simulink subsystem "GantryRobotSubsystem"  (R2024a)
settings: Solver=VariableStepAuto  StartTime=0.0  StopTime=10.0  RelTol=1e-3
model mask{DOF=3DOF, configAxis=XYZ, heightColumn=0.4, widthColumn=0.05, positionColumn1=[-0.5,-0.5,0], positionColumn2=[0.5,-0.5,0], positionColumn3=[-0.5,0.5,0], positionColumn4=[0.5,0.5,0], systemGuideX=Rail-block, strokeXMax=1, widthGuideX=0.05, diaScrewX=0.05, widthXMount=0.1, typeInertiaGuideX=Calculate from Geometry, densityGuideX=2700, massGuideX=0.1, COMGuideX=[0 0 0], MOIGuideX=[0.01 0.01 0.01], POIGuideX=[0 0 0], typeInertiaCarriageX=Calculate from Geometry, densityCarriageX=2700, massCarriageX=0.1, COMCarriageX=[0 0 0], MOICarriageX=[0.01 0.01 0.01], POICarriageX=[0 0 0], colorGuideX=[0.7 0.6 0.4], colorCarriageX=[0.5 0.5 0.9], systemGuideY=Rail-block, strokeYMax=1, widthGuideY=0.05, diaScrewY=0.05, widthYMount=0.05, typeInertiaGuideY=Calculate from Geometry, densityGuideY=2700, massGuideY=0.1, COMGuideY=[0 0 0], MOIGuideY=[0.01 0.01 0.01], POIGuideY=[0 0 0], typeInertiaCarriageY=Calculate from Geometry, densityCarriageY=2700, massCarriageY=0.1, COMCarriageY=[0 0 0], MOICarriageY=[0.01 0.01 0.01], POICarriageY=[0 0 0], colorGuideY=[0.7 0.6 0.4], colorCarriageY=[0.5 0.5 0.9], systemGuideZ=Rail-block, strokeZMax=1, widthGuideZ=0.05, diaScrewZ=0.05, shiftZAxisDown=0.02, widthZMount=0.05, typeInertiaGuideZ=Calculate from Geometry, densityGuideZ=2700, massGuideZ=0.1, COMGuideZ=[0 0 0], MOIGuideZ=[0.01 0.01 0.01], POIGuideZ=[0 0 0], typeInertiaCarriageZ=Calculate from Geometry, densityCarriageZ=2700, massCarriageZ=0.1, COMCarriageZ=[0 0 0], MOICarriageZ=[0.01 0.01 0.01], POICarriageZ=[0 0 0], colorGuideZ=[0.7 0.6 0.4], colorCarriageZ=[0.5 0.5 0.9]}
  mask prompts: DOF "Degrees of freedom"; configAxis "Axis configurations"; heightColumn "Column height (m)"; widthColumn "Column width (m)"; positionColumn1 "Column 1 position (m)"; positionColumn2 "Column 2 position (m)"; positionColumn3 "Column 3 position (m)"; positionColumn4 "Column 4 position (m)"; systemGuideX "Guide system"; strokeXMax "Maximum stroke (m)"; widthGuideX "Guide width (m)"; diaScrewX "Screw diameter (m)"; widthXMount "Mount width (m)"; typeInertiaGuideX "Inertia type"; densityGuideX "Density (kg/m^3)"; massGuideX "Mass (kg)"; COMGuideX "Center of mass (m)"; MOIGuideX "Moments of inertia (kg*m^2)"; POIGuideX "Products of inertia (kg*m^2)"; typeInertiaCarriageX "Inertia type"; densityCarriageX "Density (kg/m^3)"; massCarriageX "Mass (kg)"; COMCarriageX "Center of mass (m)"; MOICarriageX "Moments of inertia (kg*m^2)"; POICarriageX "Products of inertia (kg*m^2)"; colorGuideX "Linear guide color"; colorCarriageX "Carriage color"; systemGuideY "Guide system"; strokeYMax "Maximum stroke (m)"; widthGuideY "Guide width (m)"; diaScrewY "Screw diameter (m)"; widthYMount "Mount width (m)"; typeInertiaGuideY "Inertia type"; densityGuideY "Density (kg/m^3)"; massGuideY "Mass (kg)"; COMGuideY "Center of mass (m)"; MOIGuideY "Moments of inertia (kg*m^2)"; POIGuideY "Products of inertia (kg*m^2)"; typeInertiaCarriageY "Inertia type"; densityCarriageY "Density (kg/m^3)"; massCarriageY "Mass (kg)"; COMCarriageY "Center of mass (m)"; MOICarriageY "Moments of inertia (kg*m^2)"; POICarriageY "Products of inertia (kg*m^2)"; colorGuideY "Linear guide color"; colorCarriageY "Carriage color"; systemGuideZ "Guide system"; strokeZMax "Maximum stroke (m)"; widthGuideZ "Guide width (m)"; diaScrewZ "Screw diameter (m)"; shiftZAxisDown "Downward shift of Z-axis (m)"; widthZMount "Mount width (m)"; typeInertiaGuideZ "Inertia type"; densityGuideZ "Density (kg/m^3)"; massGuideZ "Mass (kg)"; COMGuideZ "Center of mass (m)"; MOIGuideZ "Moments of inertia (kg*m^2)"; POIGuideZ "Products of inertia (kg*m^2)"; typeInertiaCarriageZ "Inertia type"; densityCarriageZ "Density (kg/m^3)"; massCarriageZ "Mass (kg)"; COMCarriageZ "Center of mass (m)"; MOICarriageZ "Moments of inertia (kg*m^2)"; POICarriageZ "Products of inertia (kg*m^2)"; colorGuideZ "Linear guide color"; colorCarriageZ "Carriage color"
undefined symbols (not defined in the file): X, Y, Z
libraries: sm_lib x92, CartesianLib x46, nesl_utility x38
(part 1 of 4)
settings Model: Creator=abirdas  LastModifiedBy=abirdas

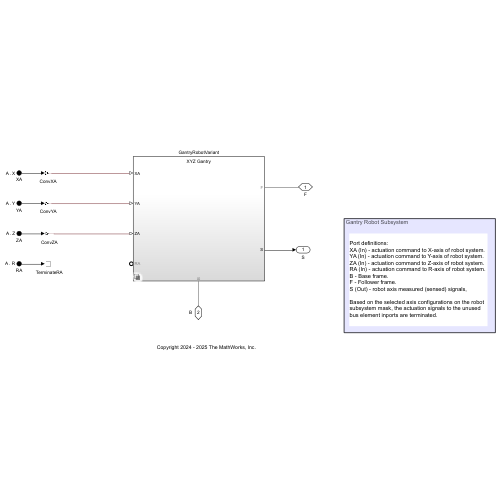
[thumbnail: Simulink's stored preview of the top-level diagram]
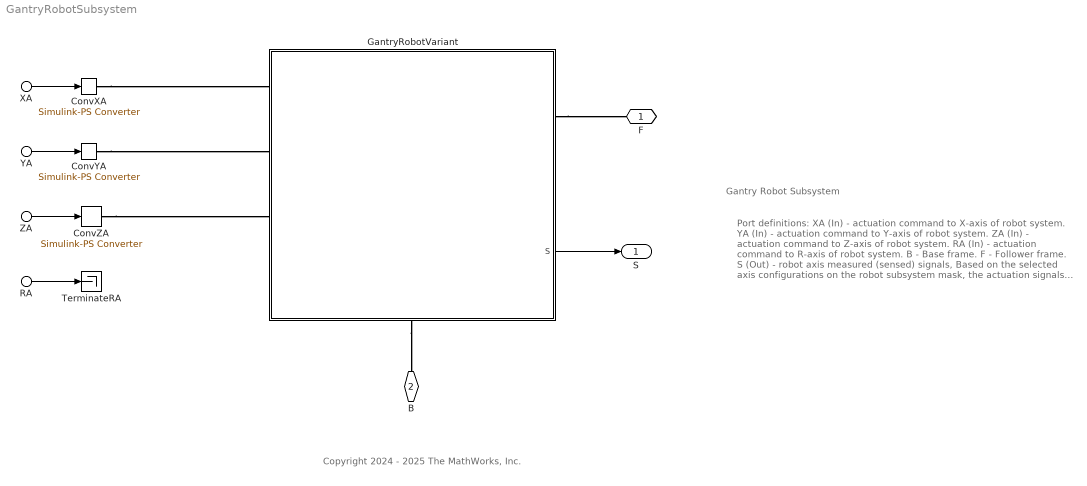
== system GantryRobotSubsystem ==
  note: Port definitions:
      | XA (In) - actuation command to X-axis of robot system.
      | YA (In) - actuation command to Y-axis of robot system.
      | ZA (In) - actuation command to Z-axis of robot system.
      | RA (In) - actuation command to R-axis of robot system.
      | B - Base frame.
      | F - Follower frame.
      | S (Out) - robot axis measured (sensed) signals,
      |
      | Based on the selected axis configurations on the robot subsystem mask, the actuation signals to the unused bus element inports are terminated.
  note: Gantry Robot Subsystem
  note: Copyright 2024 - 2025 The MathWorks, Inc.
  XA : Inport  PortName=A  Element=X
  YA : Inport  PortName=A  Element=Y
  ZA : Inport  PortName=A  Element=Z
  RA : Inport  PortName=A  Element=R
  ConvXA : nesl_utility/Simulink-PS Converter  PhysicalDomain=network_engine_domain  SubClassName=ps_input  LeftPortType=input  RightPortType=output  PseudoPeriodic=off  Frequencies=[]  NoiseDistribution=none  NoiseParameters=[]  Unit=N  AffineConversion=off  FilteringAndDerivatives=provide  SimscapeFilterOrder=1  InputFilterTimeConstant=0.001  UdotUserProvided=0
  ConvYA : nesl_utility/Simulink-PS Converter  PhysicalDomain=network_engine_domain  SubClassName=ps_input  LeftPortType=input  RightPortType=output  PseudoPeriodic=off  Frequencies=[]  NoiseDistribution=none  NoiseParameters=[]  Unit=N  AffineConversion=off  FilteringAndDerivatives=provide  SimscapeFilterOrder=1  InputFilterTimeConstant=0.001  UdotUserProvided=0
  ConvZA : nesl_utility/Simulink-PS Converter  PhysicalDomain=network_engine_domain  SubClassName=ps_input  LeftPortType=input  RightPortType=output  PseudoPeriodic=off  Frequencies=[]  NoiseDistribution=none  NoiseParameters=[]  Unit=N  AffineConversion=off  FilteringAndDerivatives=provide  SimscapeFilterOrder=1  InputFilterTimeConstant=0.001  UdotUserProvided=0
  GantryRobotVariant : Subsystem  Variant=on  VariantControlMode=label  VariantControl=Cartesian Robot  LabelModeActiveChoice=XYZG
      settings: PortSchema="{\"entries\":[{\"content\":{\"sides\":[{\"content\":{\"connectorIds\":[\"LConn1\",\"LConn2\",\"LConn3\",\"LConn4\"]},\"type\":\"ConnectorPlacement.EquallySpacedRectSide\",\"uuid\":\"05182c78-28c5-49dc-8f7f-6418cc3f9807\"},{\"content\":{\"connectorIds\":[\"RConn1\",\"Out1\"],\"side\":\"RIGHT\"},\"type\":\"ConnectorPlacement.EquallySpacedRectSide\",\"uuid\":\"f38ba8d6-0bc7-4409-a12f-2c738d3e2cd3\"},{\"content\":{\"side\":\"TOP\"},\"type\":\"ConnectorPlacement.EquallySpacedRectSide\",\"uuid\":\"c47ab8bc-feff-4301-8a81-cd6a3781eac6\"},{\"content\":{\"connectorIds\":[\"RConn2\"],\"side\":\"BOTTOM\"},\"type\":\"ConnectorPlacement.EquallySpacedRectSide\",\"uuid\":\"a09d8feb-c241-4f06-8232-e0ea8eb63063\"}]},\"type\":\"ConnectorPlacement.EquallySpacedConnector\",\"uuid\":\"47ea5a12-31cc-4b6a-9e6e-32baee4adc49\"}],\"packageUris\":[\"http://schema.mathworks.com/mf0/Connector/R2020b\"],\"version\":\"1.0\"}"
  TerminateRA : Terminator
  F : PMIOPort  Side=Right
  B : PMIOPort  Port=2  Side=Left
  S : Outport
  wires:
  GantryRobotVariant/1(S) -> S/1
  YA/1 -> ConvYA/1
  XA/1 -> ConvXA/1
  RA/1 -> TerminateRA/1
  ZA/1 -> ConvZA/1
  connections:
  GantryRobotVariant/RConn2 -- B/RConn1
  GantryRobotVariant/RConn1 -- F/RConn1
  ConvXA/RConn1 -- GantryRobotVariant/LConn1
  ConvYA/RConn1 -- GantryRobotVariant/LConn2
  ConvZA/RConn1 -- GantryRobotVariant/LConn3

== system GantryRobotSubsystem/GantryRobotVariant ==
  XY Gantry : Subsystem  VariantControl=XYG
      settings: PortSchema="{\"entries\":[{\"content\":{\"sides\":[{\"content\":{\"connectorIds\":[\"LConn1\",\"LConn2\"]},\"type\":\"ConnectorPlacement.EquallySpacedRectSide\",\"uuid\":\"0f231daf-af2e-4db7-9b9d-9d3610feb9c2\"},{\"content\":{\"connectorIds\":[\"RConn1\",\"Out1\"],\"side\":\"RIGHT\"},\"type\":\"ConnectorPlacement.EquallySpacedRectSide\",\"uuid\":\"cfb92d99-81f2-4854-933c-68fb88b1898c\"},{\"content\":{\"side\":\"TOP\"},\"type\":\"ConnectorPlacement.EquallySpacedRectSide\",\"uuid\":\"e2d61f77-b669-440a-8bc6-f5a59f9990be\"},{\"content\":{\"connectorIds\":[\"RConn2\"],\"side\":\"BOTTOM\"},\"type\":\"ConnectorPlacement.EquallySpacedRectSide\",\"uuid\":\"014f4ba7-cf54-4e14-acb9-8b5d786ed99b\"}]},\"type\":\"ConnectorPlacement.EquallySpacedConnector\",\"uuid\":\"e18480bd-7544-48c1-b55c-29c17cbfb36d\"}],\"packageUris\":[\"http://schema.mathworks.com/mf0/Connector/R2020b\"],\"version\":\"1.0\"}"
  XYZ Gantry : Subsystem  VariantControl=XYZG
      settings: PortSchema="{\"entries\":[{\"content\":{\"sides\":[{\"content\":{\"connectorIds\":[\"LConn1\",\"LConn2\",\"LConn3\"]},\"type\":\"ConnectorPlacement.EquallySpacedRectSide\",\"uuid\":\"0f231daf-af2e-4db7-9b9d-9d3610feb9c2\"},{\"content\":{\"connectorIds\":[\"RConn1\",\"Out1\"],\"side\":\"RIGHT\"},\"type\":\"ConnectorPlacement.EquallySpacedRectSide\",\"uuid\":\"cfb92d99-81f2-4854-933c-68fb88b1898c\"},{\"content\":{\"side\":\"TOP\"},\"type\":\"ConnectorPlacement.EquallySpacedRectSide\",\"uuid\":\"e2d61f77-b669-440a-8bc6-f5a59f9990be\"},{\"content\":{\"connectorIds\":[\"RConn2\"],\"side\":\"BOTTOM\"},\"type\":\"ConnectorPlacement.EquallySpacedRectSide\",\"uuid\":\"014f4ba7-cf54-4e14-acb9-8b5d786ed99b\"}]},\"type\":\"ConnectorPlacement.EquallySpacedConnector\",\"uuid\":\"e18480bd-7544-48c1-b55c-29c17cbfb36d\"}],\"packageUris\":[\"http://schema.mathworks.com/mf0/Connector/R2020b\"],\"version\":\"1.0\"}"
  XYZR Gantry : Subsystem  VariantControl=XYZRG
      settings: PortSchema="{\"entries\":[{\"content\":{\"sides\":[{\"content\":{\"connectorIds\":[\"LConn1\",\"LConn2\",\"LConn3\",\"LConn4\"]},\"type\":\"ConnectorPlacement.EquallySpacedRectSide\",\"uuid\":\"0f231daf-af2e-4db7-9b9d-9d3610feb9c2\"},{\"content\":{\"connectorIds\":[\"RConn1\",\"Out1\"],\"side\":\"RIGHT\"},\"type\":\"ConnectorPlacement.EquallySpacedRectSide\",\"uuid\":\"cfb92d99-81f2-4854-933c-68fb88b1898c\"},{\"content\":{\"side\":\"TOP\"},\"type\":\"ConnectorPlacement.EquallySpacedRectSide\",\"uuid\":\"e2d61f77-b669-440a-8bc6-f5a59f9990be\"},{\"content\":{\"connectorIds\":[\"RConn2\"],\"side\":\"BOTTOM\"},\"type\":\"ConnectorPlacement.EquallySpacedRectSide\",\"uuid\":\"014f4ba7-cf54-4e14-acb9-8b5d786ed99b\"}]},\"type\":\"ConnectorPlacement.EquallySpacedConnector\",\"uuid\":\"e18480bd-7544-48c1-b55c-29c17cbfb36d\"}],\"packageUris\":[\"http://schema.mathworks.com/mf0/Connector/R2020b\"],\"version\":\"1.0\"}"
  F : PMIOPort  Side=Right
  B : PMIOPort  Port=2  Side=Right
  XA : PMIOPort  Port=3  Side=Left
  YA : PMIOPort  Port=4  Side=Left
  ZA : PMIOPort  Port=5  Side=Left
  RA : PMIOPort  Port=6  Side=Left
  S : Outport

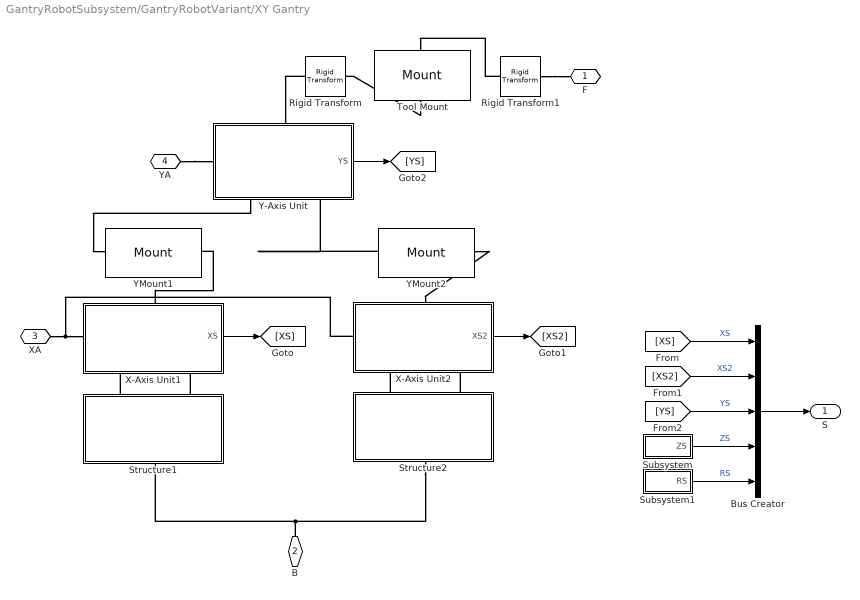
== system GantryRobotSubsystem/GantryRobotVariant/XY Gantry ==
  Bus Creator : BusCreator  Inputs=5
  Rigid Transform : sm_lib/Frames and Transforms/Rigid Transform  RotationMethod=StandardAxis  FollAlignAxisA=+X  BaseAlignAxisA=+Y  FollAlignAxisB=+Y  BaseAlignAxisB=+Z  RotationStandardAxis=+Y  RotationAngle=90  RotationAngleUnits=deg  RotationArbitraryAxis=[0 0 1]  RotationSequenceAxes=FollowerAxes  RotationSequence=XYX  RotationSequenceAngles=[0 0 0]  RotationSequenceAnglesUnits=deg  RotationMatrix=[1 0 0;0 1 0;0 0 1]  Quaternion=[1 0 0 0]  TranslationMethod=None  TranslationCartesianOffset=[0 0 0]  TranslationCartesianOffsetUnits=m  TranslationStandardAxis=+Z  TranslationStandardOffset=0  TranslationStandardOffsetUnits=m  TranslationROffset=0  TranslationROffsetUnits=m  TranslationThetaOffset=0  TranslationThetaOffsetUnits=deg  TranslationZOffset=0  TranslationZOffsetUnits=m
  Rigid Transform1 : sm_lib/Frames and Transforms/Rigid Transform  RotationMethod=RotationSequence  FollAlignAxisA=+X  BaseAlignAxisA=+Y  FollAlignAxisB=+Y  BaseAlignAxisB=+Z  RotationStandardAxis=+Y  RotationAngle=-90  RotationAngleUnits=deg  RotationArbitraryAxis=[0 0 1]  RotationSequenceAxes=BaseAxes  RotationSequence=XYZ  RotationSequenceAngles=[180 -90 180]  RotationSequenceAnglesUnits=deg  RotationMatrix=[1 0 0;0 1 0;0 0 1]  Quaternion=[1 0 0 0]  TranslationMethod=None  TranslationCartesianOffset=[0 0 0]  TranslationCartesianOffsetUnits=m  TranslationStandardAxis=+X  TranslationStandardOffset=0.1  TranslationStandardOffsetUnits=m  TranslationROffset=0  TranslationROffsetUnits=m  TranslationThetaOffset=0  TranslationThetaOffsetUnits=deg  TranslationZOffset=0  TranslationZOffsetUnits=m
  Structure1 : Subsystem
      settings: PortSchema="{\"entries\":[{\"content\":{\"sides\":[{\"content\":{},\"type\":\"ConnectorPlacement.EquallySpacedRectSide\",\"uuid\":\"5b485af5-4f05-4248-a7f3-08377bf9cff2\"},{\"content\":{\"side\":\"RIGHT\"},\"type\":\"ConnectorPlacement.EquallySpacedRectSide\",\"uuid\":\"824380b3-967b-4422-aed9-09760effc9b4\"},{\"content\":{\"connectorIds\":[\"LConn1\",\"LConn2\"],\"side\":\"TOP\"},\"type\":\"ConnectorPlacement.EquallySpacedRectSide\",\"uuid\":\"4c7d634e-a270-49ee-a9b6-ce866eb97663\"},{\"content\":{\"connectorIds\":[\"RConn1\"],\"side\":\"BOTTOM\"},\"type\":\"ConnectorPlacement.EquallySpacedRectSide\",\"uuid\":\"661dce3c-0d5e-4d43-b6d0-624fcf5b4344\"}]},\"type\":\"ConnectorPlacement.EquallySpacedConnector\",\"uuid\":\"704e5fa1-0bef-4b5b-a1a4-570354550c26\"}],\"packageUris\":[\"http://schema.mathworks.com/mf0/Connector/R2020b\"],\"version\":\"1.0\"}"
      mask Display: image('GantryStructure.png');
  Structure2 : Subsystem
      settings: PortSchema="{\"entries\":[{\"content\":{\"sides\":[{\"content\":{},\"type\":\"ConnectorPlacement.EquallySpacedRectSide\",\"uuid\":\"02cc9e51-a55a-4707-81bb-2b8bc315fd21\"},{\"content\":{\"side\":\"RIGHT\"},\"type\":\"ConnectorPlacement.EquallySpacedRectSide\",\"uuid\":\"a2e99c54-f09b-4985-a7ea-af73e820527d\"},{\"content\":{\"connectorIds\":[\"LConn1\",\"LConn2\"],\"side\":\"TOP\"},\"type\":\"ConnectorPlacement.EquallySpacedRectSide\",\"uuid\":\"28f5dd0e-9b4c-4e48-8b36-544f43ecb487\"},{\"content\":{\"connectorIds\":[\"RConn1\"],\"side\":\"BOTTOM\"},\"type\":\"ConnectorPlacement.EquallySpacedRectSide\",\"uuid\":\"f7ad5760-0a28-4c8d-8ad1-4b2be2ef73e5\"}]},\"type\":\"ConnectorPlacement.EquallySpacedConnector\",\"uuid\":\"bc63718e-7e02-41d2-9d22-b372ba5e1b36\"}],\"packageUris\":[\"http://schema.mathworks.com/mf0/Connector/R2020b\"],\"version\":\"1.0\"}"
      mask Display: image('GantryStructure.png');
  Subsystem : Subsystem
  Subsystem1 : Subsystem
  Tool Mount : CartesianLib/Mount  typeMount=Plate mount  widthMount=widthYMount  angleMount=45  angleRotate=0  typeInertiaMount=Calculate from Geometry  densityMount=2700  massMount=0.1  CMMount=[0 0 0]  MOIMount=[1 1 1]  POIMount=[0 0 0]  colorMount=[0.35 0.25 0.25]
  X-Axis Unit1 : Subsystem
      settings: PortSchema="{\"entries\":[{\"content\":{\"sides\":[{\"content\":{\"connectorIds\":[\"LConn1\"]},\"type\":\"ConnectorPlacement.EquallySpacedRectSide\",\"uuid\":\"02cc9e51-a55a-4707-81bb-2b8bc315fd21\"},{\"content\":{\"connectorIds\":[\"Out1\"],\"side\":\"RIGHT\"},\"type\":\"ConnectorPlacement.EquallySpacedRectSide\",\"uuid\":\"a2e99c54-f09b-4985-a7ea-af73e820527d\"},{\"content\":{\"connectorIds\":[\"LConn2\"],\"side\":\"TOP\"},\"type\":\"ConnectorPlacement.EquallySpacedRectSide\",\"uuid\":\"28f5dd0e-9b4c-4e48-8b36-544f43ecb487\"},{\"content\":{\"connectorIds\":[\"RConn1\",\"RConn2\"],\"side\":\"BOTTOM\"},\"type\":\"ConnectorPlacement.EquallySpacedRectSide\",\"uuid\":\"c9464558-44f4-4ab6-8590-015684f382ae\"}]},\"type\":\"ConnectorPlacement.EquallySpacedConnector\",\"uuid\":\"bc63718e-7e02-41d2-9d22-b372ba5e1b36\"}],\"packageUris\":[\"http://schema.mathworks.com/mf0/Connector/R2020b\"],\"version\":\"1.0\"}"
  X-Axis Unit2 : Subsystem
      settings: PortSchema="{\"entries\":[{\"content\":{\"sides\":[{\"content\":{\"connectorIds\":[\"LConn1\"]},\"type\":\"ConnectorPlacement.EquallySpacedRectSide\",\"uuid\":\"02cc9e51-a55a-4707-81bb-2b8bc315fd21\"},{\"content\":{\"connectorIds\":[\"Out1\"],\"side\":\"RIGHT\"},\"type\":\"ConnectorPlacement.EquallySpacedRectSide\",\"uuid\":\"a2e99c54-f09b-4985-a7ea-af73e820527d\"},{\"content\":{\"connectorIds\":[\"LConn2\"],\"side\":\"TOP\"},\"type\":\"ConnectorPlacement.EquallySpacedRectSide\",\"uuid\":\"28f5dd0e-9b4c-4e48-8b36-544f43ecb487\"},{\"content\":{\"connectorIds\":[\"RConn1\",\"RConn2\"],\"side\":\"BOTTOM\"},\"type\":\"ConnectorPlacement.EquallySpacedRectSide\",\"uuid\":\"8194e2a8-970f-447a-8fcf-69b7af47610c\"}]},\"type\":\"ConnectorPlacement.EquallySpacedConnector\",\"uuid\":\"bc63718e-7e02-41d2-9d22-b372ba5e1b36\"}],\"packageUris\":[\"http://schema.mathworks.com/mf0/Connector/R2020b\"],\"version\":\"1.0\"}"
  Y-Axis Unit : Subsystem
      settings: PortSchema="{\"entries\":[{\"content\":{\"sides\":[{\"content\":{\"connectorIds\":[\"LConn1\"]},\"type\":\"ConnectorPlacement.EquallySpacedRectSide\",\"uuid\":\"02cc9e51-a55a-4707-81bb-2b8bc315fd21\"},{\"content\":{\"connectorIds\":[\"Out1\"],\"side\":\"RIGHT\"},\"type\":\"ConnectorPlacement.EquallySpacedRectSide\",\"uuid\":\"a2e99c54-f09b-4985-a7ea-af73e820527d\"},{\"content\":{\"connectorIds\":[\"LConn2\"],\"side\":\"TOP\"},\"type\":\"ConnectorPlacement.EquallySpacedRectSide\",\"uuid\":\"28f5dd0e-9b4c-4e48-8b36-544f43ecb487\"},{\"content\":{\"connectorIds\":[\"RConn1\",\"RConn2\"],\"side\":\"BOTTOM\"},\"type\":\"ConnectorPlacement.EquallySpacedRectSide\",\"uuid\":\"d236e95f-8c0e-4e9d-a13a-e603309ee4cf\"}]},\"type\":\"ConnectorPlacement.EquallySpacedConnector\",\"uuid\":\"bc63718e-7e02-41d2-9d22-b372ba5e1b36\"}],\"packageUris\":[\"http://schema.mathworks.com/mf0/Connector/R2020b\"],\"version\":\"1.0\"}"
  YMount1 : CartesianLib/Mount  typeMount=L-shaped mount  widthMount=widthYMount  angleMount=45  angleRotate=0  typeInertiaMount=Calculate from Geometry  densityMount=2700  massMount=0.1  CMMount=[0 0 0]  MOIMount=[1 1 1]  POIMount=[0 0 0]  colorMount=[0.35 0.25 0.25]
  YMount2 : CartesianLib/Mount  typeMount=L-shaped mount  widthMount=widthYMount  angleMount=45  angleRotate=0  typeInertiaMount=Calculate from Geometry  densityMount=2700  massMount=0.1  CMMount=[0 0 0]  MOIMount=[1 1 1]  POIMount=[0 0 0]  colorMount=[0.35 0.25 0.25]
  F : PMIOPort  Side=Right
  B : PMIOPort  Port=2  Side=Right
  XA : PMIOPort  Port=3  Side=Left
  YA : PMIOPort  Port=4  Side=Left
  S : Outport
  wires:
  [XS2] -> Bus Creator/2  "XS2"
  [XS] -> Bus Creator/1  "XS"
  Bus Creator/1 -> S/1
  [YS] -> Bus Creator/3  "YS"
  Y-Axis Unit/1(YS) -> [YS]
  X-Axis Unit2/1(XS2) -> [XS2]
  X-Axis Unit1/1(XS) -> [XS]
  Subsystem/1(ZS) -> Bus Creator/4  "ZS"
  Subsystem1/1(RS) -> Bus Creator/5  "RS"
  connections:
  YA/RConn1 -- Y-Axis Unit/LConn1
  X-Axis Unit1/LConn1 -- X-Axis Unit2/LConn1 -- XA/RConn1
  Structure2/LConn2 -- X-Axis Unit2/RConn2
  Structure1/LConn2 -- X-Axis Unit1/RConn2
  Rigid Transform1/RConn1 -- F/RConn1
  Rigid Transform/LConn1 -- Y-Axis Unit/LConn2
  X-Axis Unit1/LConn2 -- YMount1/RConn1
  YMount2/RConn1 -- X-Axis Unit2/LConn2
  YMount2/LConn1 -- Y-Axis Unit/RConn2
  Structure1/RConn1 -- B/RConn1 -- Structure2/RConn1
  Structure1/LConn1 -- X-Axis Unit1/RConn1
  Structure2/LConn1 -- X-Axis Unit2/RConn1
  Tool Mount/RConn1 -- Rigid Transform/RConn1
  Y-Axis Unit/RConn1 -- YMount1/LConn1
  Rigid Transform1/LConn1 -- Tool Mount/LConn1

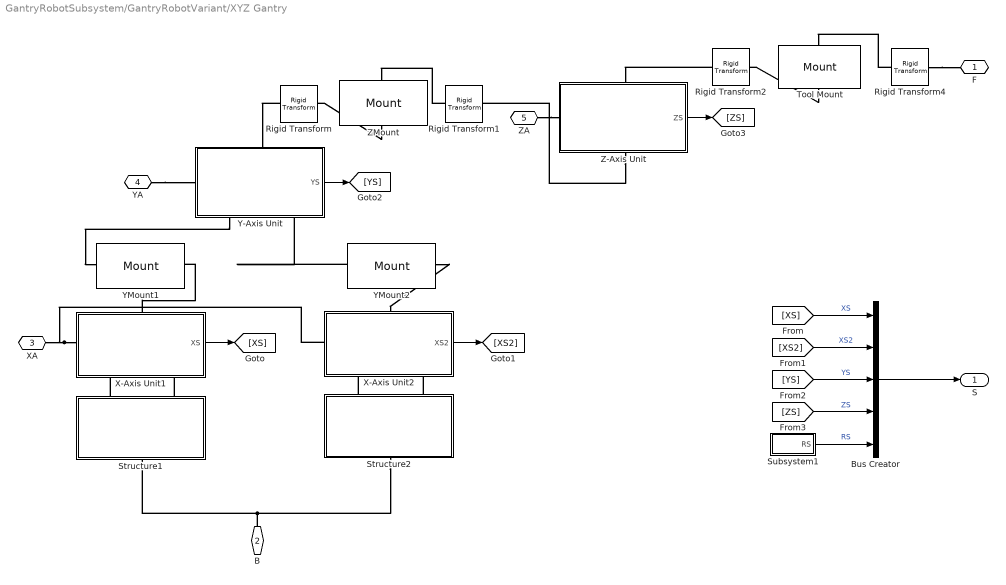
== system GantryRobotSubsystem/GantryRobotVariant/XYZ Gantry ==
  Bus Creator : BusCreator  Inputs=5
  Rigid Transform : sm_lib/Frames and Transforms/Rigid Transform  RotationMethod=StandardAxis  FollAlignAxisA=+X  BaseAlignAxisA=+Y  FollAlignAxisB=+Y  BaseAlignAxisB=+Z  RotationStandardAxis=+Y  RotationAngle=90  RotationAngleUnits=deg  RotationArbitraryAxis=[0 0 1]  RotationSequenceAxes=FollowerAxes  RotationSequence=XYX  RotationSequenceAngles=[0 0 0]  RotationSequenceAnglesUnits=deg  RotationMatrix=[1 0 0;0 1 0;0 0 1]  Quaternion=[1 0 0 0]  TranslationMethod=None  TranslationCartesianOffset=[0 0 0]  TranslationCartesianOffsetUnits=m  TranslationStandardAxis=+Z  TranslationStandardOffset=0  TranslationStandardOffsetUnits=m  TranslationROffset=0  TranslationROffsetUnits=m  TranslationThetaOffset=0  TranslationThetaOffsetUnits=deg  TranslationZOffset=0  TranslationZOffsetUnits=m
  Rigid Transform1 : sm_lib/Frames and Transforms/Rigid Transform  RotationMethod=RotationSequence  FollAlignAxisA=+X  BaseAlignAxisA=+Y  FollAlignAxisB=+Y  BaseAlignAxisB=+Z  RotationStandardAxis=+Y  RotationAngle=-90  RotationAngleUnits=deg  RotationArbitraryAxis=[0 0 1]  RotationSequenceAxes=BaseAxes  RotationSequence=XYZ  RotationSequenceAngles=[0 -90 180]  RotationSequenceAnglesUnits=deg  RotationMatrix=[1 0 0;0 1 0;0 0 1]  Quaternion=[1 0 0 0]  TranslationMethod=None  TranslationCartesianOffset=[0 0 0]  TranslationCartesianOffsetUnits=m  TranslationStandardAxis=+X  TranslationStandardOffset=0.1  TranslationStandardOffsetUnits=m  TranslationROffset=0  TranslationROffsetUnits=m  TranslationThetaOffset=0  TranslationThetaOffsetUnits=deg  TranslationZOffset=0  TranslationZOffsetUnits=m
  Rigid Transform2 : sm_lib/Frames and Transforms/Rigid Transform  RotationMethod=RotationSequence  FollAlignAxisA=+X  BaseAlignAxisA=+Y  FollAlignAxisB=+Y  BaseAlignAxisB=+Z  RotationStandardAxis=+X  RotationAngle=180  RotationAngleUnits=deg  RotationArbitraryAxis=[0 0 1]  RotationSequenceAxes=BaseAxes  RotationSequence=XYZ  RotationSequenceAngles=[180 -90 0]  RotationSequenceAnglesUnits=deg  RotationMatrix=[1 0 0;0 1 0;0 0 1]  Quaternion=[1 0 0 0]  TranslationMethod=None  TranslationCartesianOffset=[0 0 0]  TranslationCartesianOffsetUnits=m  TranslationStandardAxis=+Z  TranslationStandardOffset=0  TranslationStandardOffsetUnits=m  TranslationROffset=0  TranslationROffsetUnits=m  TranslationThetaOffset=0  TranslationThetaOffsetUnits=deg  TranslationZOffset=0  TranslationZOffsetUnits=m
  Rigid Transform4 : sm_lib/Frames and Transforms/Rigid Transform  RotationMethod=StandardAxis  FollAlignAxisA=+X  BaseAlignAxisA=+Y  FollAlignAxisB=+Y  BaseAlignAxisB=+Z  RotationStandardAxis=+Y  RotationAngle=-90  RotationAngleUnits=deg  RotationArbitraryAxis=[0 0 1]  RotationSequenceAxes=FollowerAxes  RotationSequence=XYX  RotationSequenceAngles=[0 0 0]  RotationSequenceAnglesUnits=deg  RotationMatrix=[1 0 0;0 1 0;0 0 1]  Quaternion=[1 0 0 0]  TranslationMethod=None  TranslationCartesianOffset=[0 0 0]  TranslationCartesianOffsetUnits=m  TranslationStandardAxis=+X  TranslationStandardOffset=0.1  TranslationStandardOffsetUnits=m  TranslationROffset=0  TranslationROffsetUnits=m  TranslationThetaOffset=0  TranslationThetaOffsetUnits=deg  TranslationZOffset=0  TranslationZOffsetUnits=m
  Structure1 : Subsystem
      settings: PortSchema="{\"entries\":[{\"content\":{\"sides\":[{\"content\":{},\"type\":\"ConnectorPlacement.EquallySpacedRectSide\",\"uuid\":\"5b485af5-4f05-4248-a7f3-08377bf9cff2\"},{\"content\":{\"side\":\"RIGHT\"},\"type\":\"ConnectorPlacement.EquallySpacedRectSide\",\"uuid\":\"824380b3-967b-4422-aed9-09760effc9b4\"},{\"content\":{\"connectorIds\":[\"LConn1\",\"LConn2\"],\"side\":\"TOP\"},\"type\":\"ConnectorPlacement.EquallySpacedRectSide\",\"uuid\":\"4c7d634e-a270-49ee-a9b6-ce866eb97663\"},{\"content\":{\"connectorIds\":[\"RConn1\"],\"side\":\"BOTTOM\"},\"type\":\"ConnectorPlacement.EquallySpacedRectSide\",\"uuid\":\"661dce3c-0d5e-4d43-b6d0-624fcf5b4344\"}]},\"type\":\"ConnectorPlacement.EquallySpacedConnector\",\"uuid\":\"704e5fa1-0bef-4b5b-a1a4-570354550c26\"}],\"packageUris\":[\"http://schema.mathworks.com/mf0/Connector/R2020b\"],\"version\":\"1.0\"}"
      mask Display: image('GantryStructure.png');
  Structure2 : Subsystem
      settings: PortSchema="{\"entries\":[{\"content\":{\"sides\":[{\"content\":{},\"type\":\"ConnectorPlacement.EquallySpacedRectSide\",\"uuid\":\"02cc9e51-a55a-4707-81bb-2b8bc315fd21\"},{\"content\":{\"side\":\"RIGHT\"},\"type\":\"ConnectorPlacement.EquallySpacedRectSide\",\"uuid\":\"a2e99c54-f09b-4985-a7ea-af73e820527d\"},{\"content\":{\"connectorIds\":[\"LConn1\",\"LConn2\"],\"side\":\"TOP\"},\"type\":\"ConnectorPlacement.EquallySpacedRectSide\",\"uuid\":\"28f5dd0e-9b4c-4e48-8b36-544f43ecb487\"},{\"content\":{\"connectorIds\":[\"RConn1\"],\"side\":\"BOTTOM\"},\"type\":\"ConnectorPlacement.EquallySpacedRectSide\",\"uuid\":\"f7ad5760-0a28-4c8d-8ad1-4b2be2ef73e5\"}]},\"type\":\"ConnectorPlacement.EquallySpacedConnector\",\"uuid\":\"bc63718e-7e02-41d2-9d22-b372ba5e1b36\"}],\"packageUris\":[\"http://schema.mathworks.com/mf0/Connector/R2020b\"],\"version\":\"1.0\"}"
      mask Display: image('GantryStructure.png');
  Subsystem1 : Subsystem
  Tool Mount : CartesianLib/Mount  typeMount=Plate mount  widthMount=widthZMount  angleMount=45  angleRotate=0  typeInertiaMount=Calculate from Geometry  densityMount=2700  massMount=0.1  CMMount=[0 0 0]  MOIMount=[1 1 1]  POIMount=[0 0 0]  colorMount=[0.35 0.25 0.25]
  X-Axis Unit1 : Subsystem
      settings: PortSchema="{\"entries\":[{\"content\":{\"sides\":[{\"content\":{\"connectorIds\":[\"LConn1\"]},\"type\":\"ConnectorPlacement.EquallySpacedRectSide\",\"uuid\":\"02cc9e51-a55a-4707-81bb-2b8bc315fd21\"},{\"content\":{\"connectorIds\":[\"Out1\"],\"side\":\"RIGHT\"},\"type\":\"ConnectorPlacement.EquallySpacedRectSide\",\"uuid\":\"a2e99c54-f09b-4985-a7ea-af73e820527d\"},{\"content\":{\"connectorIds\":[\"LConn2\"],\"side\":\"TOP\"},\"type\":\"ConnectorPlacement.EquallySpacedRectSide\",\"uuid\":\"28f5dd0e-9b4c-4e48-8b36-544f43ecb487\"},{\"content\":{\"connectorIds\":[\"RConn1\",\"RConn2\"],\"side\":\"BOTTOM\"},\"type\":\"ConnectorPlacement.EquallySpacedRectSide\",\"uuid\":\"c9464558-44f4-4ab6-8590-015684f382ae\"}]},\"type\":\"ConnectorPlacement.EquallySpacedConnector\",\"uuid\":\"bc63718e-7e02-41d2-9d22-b372ba5e1b36\"}],\"packageUris\":[\"http://schema.mathworks.com/mf0/Connector/R2020b\"],\"version\":\"1.0\"}"
  X-Axis Unit2 : Subsystem
      settings: PortSchema="{\"entries\":[{\"content\":{\"sides\":[{\"content\":{\"connectorIds\":[\"LConn1\"]},\"type\":\"ConnectorPlacement.EquallySpacedRectSide\",\"uuid\":\"02cc9e51-a55a-4707-81bb-2b8bc315fd21\"},{\"content\":{\"connectorIds\":[\"Out1\"],\"side\":\"RIGHT\"},\"type\":\"ConnectorPlacement.EquallySpacedRectSide\",\"uuid\":\"a2e99c54-f09b-4985-a7ea-af73e820527d\"},{\"content\":{\"connectorIds\":[\"LConn2\"],\"side\":\"TOP\"},\"type\":\"ConnectorPlacement.EquallySpacedRectSide\",\"uuid\":\"28f5dd0e-9b4c-4e48-8b36-544f43ecb487\"},{\"content\":{\"connectorIds\":[\"RConn1\",\"RConn2\"],\"side\":\"BOTTOM\"},\"type\":\"ConnectorPlacement.EquallySpacedRectSide\",\"uuid\":\"8194e2a8-970f-447a-8fcf-69b7af47610c\"}]},\"type\":\"ConnectorPlacement.EquallySpacedConnector\",\"uuid\":\"bc63718e-7e02-41d2-9d22-b372ba5e1b36\"}],\"packageUris\":[\"http://schema.mathworks.com/mf0/Connector/R2020b\"],\"version\":\"1.0\"}"
  Y-Axis Unit : Subsystem
      settings: PortSchema="{\"entries\":[{\"content\":{\"sides\":[{\"content\":{\"connectorIds\":[\"LConn1\"]},\"type\":\"ConnectorPlacement.EquallySpacedRectSide\",\"uuid\":\"02cc9e51-a55a-4707-81bb-2b8bc315fd21\"},{\"content\":{\"connectorIds\":[\"Out1\"],\"side\":\"RIGHT\"},\"type\":\"ConnectorPlacement.EquallySpacedRectSide\",\"uuid\":\"a2e99c54-f09b-4985-a7ea-af73e820527d\"},{\"content\":{\"connectorIds\":[\"LConn2\"],\"side\":\"TOP\"},\"type\":\"ConnectorPlacement.EquallySpacedRectSide\",\"uuid\":\"28f5dd0e-9b4c-4e48-8b36-544f43ecb487\"},{\"content\":{\"connectorIds\":[\"RConn1\",\"RConn2\"],\"side\":\"BOTTOM\"},\"type\":\"ConnectorPlacement.EquallySpacedRectSide\",\"uuid\":\"d236e95f-8c0e-4e9d-a13a-e603309ee4cf\"}]},\"type\":\"ConnectorPlacement.EquallySpacedConnector\",\"uuid\":\"bc63718e-7e02-41d2-9d22-b372ba5e1b36\"}],\"packageUris\":[\"http://schema.mathworks.com/mf0/Connector/R2020b\"],\"version\":\"1.0\"}"
  YMount1 : CartesianLib/Mount  typeMount=L-shaped mount  widthMount=widthYMount  angleMount=45  angleRotate=0  typeInertiaMount=Calculate from Geometry  densityMount=2700  massMount=0.1  CMMount=[0 0 0]  MOIMount=[1 1 1]  POIMount=[0 0 0]  colorMount=[0.35 0.25 0.25]
  YMount2 : CartesianLib/Mount  typeMount=L-shaped mount  widthMount=widthYMount  angleMount=45  angleRotate=0  typeInertiaMount=Calculate from Geometry  densityMount=2700  massMount=0.1  CMMount=[0 0 0]  MOIMount=[1 1 1]  POIMount=[0 0 0]  colorMount=[0.35 0.25 0.25]
  Z-Axis Unit : Subsystem
      settings: PortSchema="{\"entries\":[{\"content\":{\"sides\":[{\"content\":{\"connectorIds\":[\"LConn1\"]},\"type\":\"ConnectorPlacement.EquallySpacedRectSide\",\"uuid\":\"02cc9e51-a55a-4707-81bb-2b8bc315fd21\"},{\"content\":{\"connectorIds\":[\"Out1\"],\"side\":\"RIGHT\"},\"type\":\"ConnectorPlacement.EquallySpacedRectSide\",\"uuid\":\"a2e99c54-f09b-4985-a7ea-af73e820527d\"},{\"content\":{\"connectorIds\":[\"LConn2\"],\"side\":\"TOP\"},\"type\":\"ConnectorPlacement.EquallySpacedRectSide\",\"uuid\":\"28f5dd0e-9b4c-4e48-8b36-544f43ecb487\"},{\"content\":{\"connectorIds\":[\"RConn1\"],\"side\":\"BOTTOM\"},\"type\":\"ConnectorPlacement.EquallySpacedRectSide\",\"uuid\":\"d236e95f-8c0e-4e9d-a13a-e603309ee4cf\"}]},\"type\":\"ConnectorPlacement.EquallySpacedConnector\",\"uuid\":\"bc63718e-7e02-41d2-9d22-b372ba5e1b36\"}],\"packageUris\":[\"http://schema.mathworks.com/mf0/Connector/R2020b\"],\"version\":\"1.0\"}"
  ZMount : CartesianLib/Mount  typeMount=Plate mount  widthMount=widthZMount  angleMount=45  angleRotate=0  typeInertiaMount=Calculate from Geometry  densityMount=2700  massMount=0.1  CMMount=[0 0 0]  MOIMount=[1 1 1]  POIMount=[0 0 0]  colorMount=[0.35 0.25 0.25]
  F : PMIOPort  Side=Right
  B : PMIOPort  Port=2  Side=Right
  XA : PMIOPort  Port=3  Side=Left
  YA : PMIOPort  Port=4  Side=Left
  ZA : PMIOPort  Port=5  Side=Left
  S : Outport
  wires:
  Bus Creator/1 -> S/1
  [ZS] -> Bus Creator/4  "ZS"
  [YS] -> Bus Creator/3  "YS"
  [XS2] -> Bus Creator/2  "XS2"
  [XS] -> Bus Creator/1  "XS"
  Z-Axis Unit/1(ZS) -> [ZS]
  Y-Axis Unit/1(YS) -> [YS]
  X-Axis Unit2/1(XS2) -> [XS2]
  X-Axis Unit1/1(XS) -> [XS]
  Subsystem1/1(RS) -> Bus Creator/5  "RS"
  connections:
  ZA/RConn1 -- Z-Axis Unit/LConn1
  YA/RConn1 -- Y-Axis Unit/LConn1
  X-Axis Unit1/LConn1 -- X-Axis Unit2/LConn1 -- XA/RConn1
  Structure2/LConn2 -- X-Axis Unit2/RConn2
  Structure1/LConn2 -- X-Axis Unit1/RConn2
  Rigid Transform4/RConn1 -- F/RConn1
  Tool Mount/RConn1 -- Rigid Transform2/RConn1
  Rigid Transform4/LConn1 -- Tool Mount/LConn1
  Rigid Transform/LConn1 -- Y-Axis Unit/LConn2
  X-Axis Unit1/LConn2 -- YMount1/RConn1
  Rigid Transform2/LConn1 -- Z-Axis Unit/LConn2
  YMount2/RConn1 -- X-Axis Unit2/LConn2
  YMount2/LConn1 -- Y-Axis Unit/RConn2
  Structure2/RConn1 -- B/RConn1 -- Structure1/RConn1
  Structure1/LConn1 -- X-Axis Unit1/RConn1
  Structure2/LConn1 -- X-Axis Unit2/RConn1
  Z-Axis Unit/RConn1 -- Rigid Transform1/RConn1
  ZMount/RConn1 -- Rigid Transform/RConn1
  Y-Axis Unit/RConn1 -- YMount1/LConn1
  Rigid Transform1/LConn1 -- ZMount/LConn1

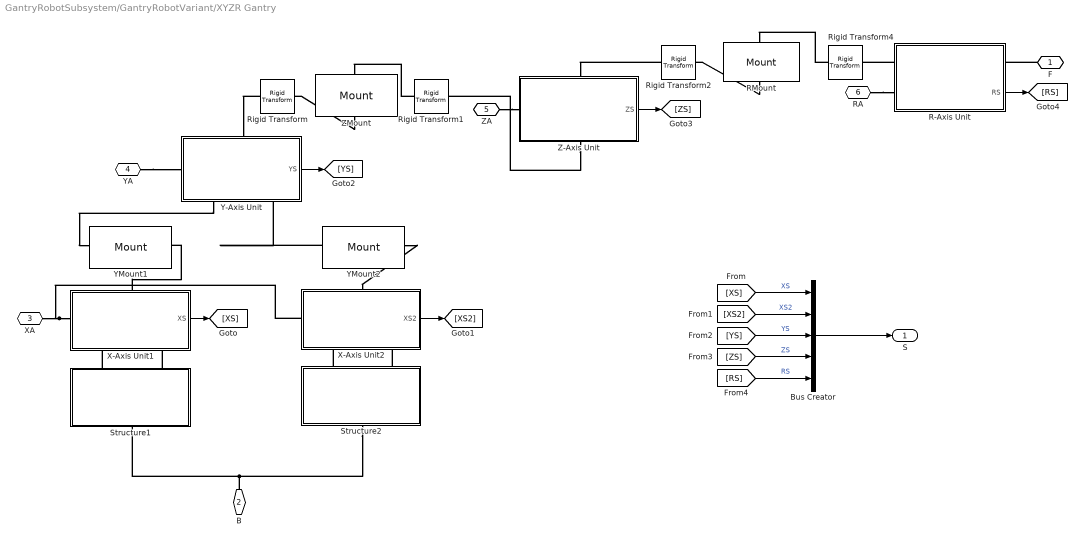
== system GantryRobotSubsystem/GantryRobotVariant/XYZR Gantry ==
  Bus Creator : BusCreator  Inputs=5
  R-Axis Unit : Subsystem
      settings: PortSchema="{\"entries\":[{\"content\":{\"sides\":[{\"content\":{\"connectorIds\":[\"LConn1\",\"LConn2\"]},\"type\":\"ConnectorPlacement.EquallySpacedRectSide\",\"uuid\":\"12736c12-94fc-4c1e-a447-e3bd5b68bdbc\"},{\"content\":{\"connectorIds\":[\"RConn1\",\"Out1\"],\"side\":\"RIGHT\"},\"type\":\"ConnectorPlacement.EquallySpacedRectSide\",\"uuid\":\"44150b67-8c91-4bb2-9a6c-3dcf829287cb\"},{\"content\":{\"side\":\"TOP\"},\"type\":\"ConnectorPlacement.EquallySpacedRectSide\",\"uuid\":\"ab2669bb-9431-4ae0-b5e4-5aa5d9eee7a9\"}]},\"type\":\"ConnectorPlacement.EquallySpacedConnector\",\"uuid\":\"369e6d0b-b949-4fc0-a0da-9b8605116d15\"}],\"packageUris\":[\"http://schema.mathworks.com/mf0/Connector/R2020b\"],\"version\":\"1.0\"}"
  RMount : CartesianLib/Mount  typeMount=Plate mount  widthMount=widthZMount  angleMount=45  angleRotate=0  typeInertiaMount=Calculate from Geometry  densityMount=2700  massMount=0.1  CMMount=[0 0 0]  MOIMount=[1 1 1]  POIMount=[0 0 0]  colorMount=[0.35 0.25 0.25]
  Rigid Transform : sm_lib/Frames and Transforms/Rigid Transform  RotationMethod=StandardAxis  FollAlignAxisA=+X  BaseAlignAxisA=+Y  FollAlignAxisB=+Y  BaseAlignAxisB=+Z  RotationStandardAxis=+Y  RotationAngle=90  RotationAngleUnits=deg  RotationArbitraryAxis=[0 0 1]  RotationSequenceAxes=FollowerAxes  RotationSequence=XYX  RotationSequenceAngles=[0 0 0]  RotationSequenceAnglesUnits=deg  RotationMatrix=[1 0 0;0 1 0;0 0 1]  Quaternion=[1 0 0 0]  TranslationMethod=None  TranslationCartesianOffset=[0 0 0]  TranslationCartesianOffsetUnits=m  TranslationStandardAxis=+Z  TranslationStandardOffset=0  TranslationStandardOffsetUnits=m  TranslationROffset=0  TranslationROffsetUnits=m  TranslationThetaOffset=0  TranslationThetaOffsetUnits=deg  TranslationZOffset=0  TranslationZOffsetUnits=m
  Rigid Transform1 : sm_lib/Frames and Transforms/Rigid Transform  RotationMethod=RotationSequence  FollAlignAxisA=+X  BaseAlignAxisA=+Y  FollAlignAxisB=+Y  BaseAlignAxisB=+Z  RotationStandardAxis=+Y  RotationAngle=-90  RotationAngleUnits=deg  RotationArbitraryAxis=[0 0 1]  RotationSequenceAxes=BaseAxes  RotationSequence=XYZ  RotationSequenceAngles=[0 -90 180]  RotationSequenceAnglesUnits=deg  RotationMatrix=[1 0 0;0 1 0;0 0 1]  Quaternion=[1 0 0 0]  TranslationMethod=None  TranslationCartesianOffset=[0 0 0]  TranslationCartesianOffsetUnits=m  TranslationStandardAxis=+X  TranslationStandardOffset=0.1  TranslationStandardOffsetUnits=m  TranslationROffset=0  TranslationROffsetUnits=m  TranslationThetaOffset=0  TranslationThetaOffsetUnits=deg  TranslationZOffset=0  TranslationZOffsetUnits=m
  Rigid Transform2 : sm_lib/Frames and Transforms/Rigid Transform  RotationMethod=RotationSequence  FollAlignAxisA=+X  BaseAlignAxisA=+Y  FollAlignAxisB=+Y  BaseAlignAxisB=+Z  RotationStandardAxis=+X  RotationAngle=180  RotationAngleUnits=deg  RotationArbitraryAxis=[0 0 1]  RotationSequenceAxes=BaseAxes  RotationSequence=XYZ  RotationSequenceAngles=[180 -90 0]  RotationSequenceAnglesUnits=deg  RotationMatrix=[1 0 0;0 1 0;0 0 1]  Quaternion=[1 0 0 0]  TranslationMethod=None  TranslationCartesianOffset=[0 0 0]  TranslationCartesianOffsetUnits=m  TranslationStandardAxis=+Z  TranslationStandardOffset=0  TranslationStandardOffsetUnits=m  TranslationROffset=0  TranslationROffsetUnits=m  TranslationThetaOffset=0  TranslationThetaOffsetUnits=deg  TranslationZOffset=0  TranslationZOffsetUnits=m
  Rigid Transform4 : sm_lib/Frames and Transforms/Rigid Transform  RotationMethod=StandardAxis  FollAlignAxisA=+X  BaseAlignAxisA=+Y  FollAlignAxisB=+Y  BaseAlignAxisB=+Z  RotationStandardAxis=+Y  RotationAngle=-90  RotationAngleUnits=deg  RotationArbitraryAxis=[0 0 1]  RotationSequenceAxes=FollowerAxes  RotationSequence=XYX  RotationSequenceAngles=[0 0 0]  RotationSequenceAnglesUnits=deg  RotationMatrix=[1 0 0;0 1 0;0 0 1]  Quaternion=[1 0 0 0]  TranslationMethod=None  TranslationCartesianOffset=[0 0 0]  TranslationCartesianOffsetUnits=m  TranslationStandardAxis=+X  TranslationStandardOffset=0.1  TranslationStandardOffsetUnits=m  TranslationROffset=0  TranslationROffsetUnits=m  TranslationThetaOffset=0  TranslationThetaOffsetUnits=deg  TranslationZOffset=0  TranslationZOffsetUnits=m
  Structure1 : Subsystem
      settings: PortSchema="{\"entries\":[{\"content\":{\"sides\":[{\"content\":{},\"type\":\"ConnectorPlacement.EquallySpacedRectSide\",\"uuid\":\"5b485af5-4f05-4248-a7f3-08377bf9cff2\"},{\"content\":{\"side\":\"RIGHT\"},\"type\":\"ConnectorPlacement.EquallySpacedRectSide\",\"uuid\":\"824380b3-967b-4422-aed9-09760effc9b4\"},{\"content\":{\"connectorIds\":[\"LConn1\",\"LConn2\"],\"side\":\"TOP\"},\"type\":\"ConnectorPlacement.EquallySpacedRectSide\",\"uuid\":\"4c7d634e-a270-49ee-a9b6-ce866eb97663\"},{\"content\":{\"connectorIds\":[\"RConn1\"],\"side\":\"BOTTOM\"},\"type\":\"ConnectorPlacement.EquallySpacedRectSide\",\"uuid\":\"661dce3c-0d5e-4d43-b6d0-624fcf5b4344\"}]},\"type\":\"ConnectorPlacement.EquallySpacedConnector\",\"uuid\":\"704e5fa1-0bef-4b5b-a1a4-570354550c26\"}],\"packageUris\":[\"http://schema.mathworks.com/mf0/Connector/R2020b\"],\"version\":\"1.0\"}"
      mask Display: image('GantryStructure.png');
  Structure2 : Subsystem
      settings: PortSchema="{\"entries\":[{\"content\":{\"sides\":[{\"content\":{},\"type\":\"ConnectorPlacement.EquallySpacedRectSide\",\"uuid\":\"02cc9e51-a55a-4707-81bb-2b8bc315fd21\"},{\"content\":{\"side\":\"RIGHT\"},\"type\":\"ConnectorPlacement.EquallySpacedRectSide\",\"uuid\":\"a2e99c54-f09b-4985-a7ea-af73e820527d\"},{\"content\":{\"connectorIds\":[\"LConn1\",\"LConn2\"],\"side\":\"TOP\"},\"type\":\"ConnectorPlacement.EquallySpacedRectSide\",\"uuid\":\"28f5dd0e-9b4c-4e48-8b36-544f43ecb487\"},{\"content\":{\"connectorIds\":[\"RConn1\"],\"side\":\"BOTTOM\"},\"type\":\"ConnectorPlacement.EquallySpacedRectSide\",\"uuid\":\"f7ad5760-0a28-4c8d-8ad1-4b2be2ef73e5\"}]},\"type\":\"ConnectorPlacement.EquallySpacedConnector\",\"uuid\":\"bc63718e-7e02-41d2-9d22-b372ba5e1b36\"}],\"packageUris\":[\"http://schema.mathworks.com/mf0/Connector/R2020b\"],\"version\":\"1.0\"}"
      mask Display: image('GantryStructure.png');
  X-Axis Unit1 : Subsystem
      settings: PortSchema="{\"entries\":[{\"content\":{\"sides\":[{\"content\":{\"connectorIds\":[\"LConn1\"]},\"type\":\"ConnectorPlacement.EquallySpacedRectSide\",\"uuid\":\"02cc9e51-a55a-4707-81bb-2b8bc315fd21\"},{\"content\":{\"connectorIds\":[\"Out1\"],\"side\":\"RIGHT\"},\"type\":\"ConnectorPlacement.EquallySpacedRectSide\",\"uuid\":\"a2e99c54-f09b-4985-a7ea-af73e820527d\"},{\"content\":{\"connectorIds\":[\"LConn2\"],\"side\":\"TOP\"},\"type\":\"ConnectorPlacement.EquallySpacedRectSide\",\"uuid\":\"28f5dd0e-9b4c-4e48-8b36-544f43ecb487\"},{\"content\":{\"connectorIds\":[\"RConn1\",\"RConn2\"],\"side\":\"BOTTOM\"},\"type\":\"ConnectorPlacement.EquallySpacedRectSide\",\"uuid\":\"c9464558-44f4-4ab6-8590-015684f382ae\"}]},\"type\":\"ConnectorPlacement.EquallySpacedConnector\",\"uuid\":\"bc63718e-7e02-41d2-9d22-b372ba5e1b36\"}],\"packageUris\":[\"http://schema.mathworks.com/mf0/Connector/R2020b\"],\"version\":\"1.0\"}"
  X-Axis Unit2 : Subsystem
      settings: PortSchema="{\"entries\":[{\"content\":{\"sides\":[{\"content\":{\"connectorIds\":[\"LConn1\"]},\"type\":\"ConnectorPlacement.EquallySpacedRectSide\",\"uuid\":\"02cc9e51-a55a-4707-81bb-2b8bc315fd21\"},{\"content\":{\"connectorIds\":[\"Out1\"],\"side\":\"RIGHT\"},\"type\":\"ConnectorPlacement.EquallySpacedRectSide\",\"uuid\":\"a2e99c54-f09b-4985-a7ea-af73e820527d\"},{\"content\":{\"connectorIds\":[\"LConn2\"],\"side\":\"TOP\"},\"type\":\"ConnectorPlacement.EquallySpacedRectSide\",\"uuid\":\"28f5dd0e-9b4c-4e48-8b36-544f43ecb487\"},{\"content\":{\"connectorIds\":[\"RConn1\",\"RConn2\"],\"side\":\"BOTTOM\"},\"type\":\"ConnectorPlacement.EquallySpacedRectSide\",\"uuid\":\"8194e2a8-970f-447a-8fcf-69b7af47610c\"}]},\"type\":\"ConnectorPlacement.EquallySpacedConnector\",\"uuid\":\"bc63718e-7e02-41d2-9d22-b372ba5e1b36\"}],\"packageUris\":[\"http://schema.mathworks.com/mf0/Connector/R2020b\"],\"version\":\"1.0\"}"
  Y-Axis Unit : Subsystem
      settings: PortSchema="{\"entries\":[{\"content\":{\"sides\":[{\"content\":{\"connectorIds\":[\"LConn1\"]},\"type\":\"ConnectorPlacement.EquallySpacedRectSide\",\"uuid\":\"02cc9e51-a55a-4707-81bb-2b8bc315fd21\"},{\"content\":{\"connectorIds\":[\"Out1\"],\"side\":\"RIGHT\"},\"type\":\"ConnectorPlacement.EquallySpacedRectSide\",\"uuid\":\"a2e99c54-f09b-4985-a7ea-af73e820527d\"},{\"content\":{\"connectorIds\":[\"LConn2\"],\"side\":\"TOP\"},\"type\":\"ConnectorPlacement.EquallySpacedRectSide\",\"uuid\":\"28f5dd0e-9b4c-4e48-8b36-544f43ecb487\"},{\"content\":{\"connectorIds\":[\"RConn1\",\"RConn2\"],\"side\":\"BOTTOM\"},\"type\":\"ConnectorPlacement.EquallySpacedRectSide\",\"uuid\":\"d236e95f-8c0e-4e9d-a13a-e603309ee4cf\"}]},\"type\":\"ConnectorPlacement.EquallySpacedConnector\",\"uuid\":\"bc63718e-7e02-41d2-9d22-b372ba5e1b36\"}],\"packageUris\":[\"http://schema.mathworks.com/mf0/Connector/R2020b\"],\"version\":\"1.0\"}"
  YMount1 : CartesianLib/Mount  typeMount=L-shaped mount  widthMount=widthYMount  angleMount=45  angleRotate=0  typeInertiaMount=Calculate from Geometry  densityMount=2700  massMount=0.1  CMMount=[0 0 0]  MOIMount=[1 1 1]  POIMount=[0 0 0]  colorMount=[0.35 0.25 0.25]
  YMount2 : CartesianLib/Mount  typeMount=L-shaped mount  widthMount=widthYMount  angleMount=45  angleRotate=0  typeInertiaMount=Calculate from Geometry  densityMount=2700  massMount=0.1  CMMount=[0 0 0]  MOIMount=[1 1 1]  POIMount=[0 0 0]  colorMount=[0.35 0.25 0.25]
  Z-Axis Unit : Subsystem
      settings: PortSchema="{\"entries\":[{\"content\":{\"sides\":[{\"content\":{\"connectorIds\":[\"LConn1\"]},\"type\":\"ConnectorPlacement.EquallySpacedRectSide\",\"uuid\":\"02cc9e51-a55a-4707-81bb-2b8bc315fd21\"},{\"content\":{\"connectorIds\":[\"Out1\"],\"side\":\"RIGHT\"},\"type\":\"ConnectorPlacement.EquallySpacedRectSide\",\"uuid\":\"a2e99c54-f09b-4985-a7ea-af73e820527d\"},{\"content\":{\"connectorIds\":[\"LConn2\"],\"side\":\"TOP\"},\"type\":\"ConnectorPlacement.EquallySpacedRectSide\",\"uuid\":\"28f5dd0e-9b4c-4e48-8b36-544f43ecb487\"},{\"content\":{\"connectorIds\":[\"RConn1\"],\"side\":\"BOTTOM\"},\"type\":\"ConnectorPlacement.EquallySpacedRectSide\",\"uuid\":\"d236e95f-8c0e-4e9d-a13a-e603309ee4cf\"}]},\"type\":\"ConnectorPlacement.EquallySpacedConnector\",\"uuid\":\"bc63718e-7e02-41d2-9d22-b372ba5e1b36\"}],\"packageUris\":[\"http://schema.mathworks.com/mf0/Connector/R2020b\"],\"version\":\"1.0\"}"
  ZMount : CartesianLib/Mount  typeMount=Plate mount  widthMount=widthZMount  angleMount=45  angleRotate=0  typeInertiaMount=Calculate from Geometry  densityMount=2700  massMount=0.1  CMMount=[0 0 0]  MOIMount=[1 1 1]  POIMount=[0 0 0]  colorMount=[0.35 0.25 0.25]
  F : PMIOPort  Side=Right
  B : PMIOPort  Port=2  Side=Right
  XA : PMIOPort  Port=3  Side=Left
  YA : PMIOPort  Port=4  Side=Left
  ZA : PMIOPort  Port=5  Side=Left
  RA : PMIOPort  Port=6  Side=Left
  S : Outport
  wires:
  Bus Creator/1 -> S/1
  [ZS] -> Bus Creator/4  "ZS"
  [YS] -> Bus Creator/3  "YS"
  [XS2] -> Bus Creator/2  "XS2"
  [XS] -> Bus Creator/1  "XS"
  Z-Axis Unit/1(ZS) -> [ZS]
  Y-Axis Unit/1(YS) -> [YS]
  X-Axis Unit2/1(XS2) -> [XS2]
  X-Axis Unit1/1(XS) -> [XS]
  R-Axis Unit/1(RS) -> [RS]
  [RS] -> Bus Creator/5  "RS"
  connections:
  ZA/RConn1 -- Z-Axis Unit/LConn1
  YA/RConn1 -- Y-Axis Unit/LConn1
  X-Axis Unit1/LConn1 -- X-Axis Unit2/LConn1 -- XA/RConn1
  Structure2/LConn2 -- X-Axis Unit2/RConn2
  Structure1/LConn2 -- X-Axis Unit1/RConn2
  RMount/RConn1 -- Rigid Transform2/RConn1
  Rigid Transform4/LConn1 -- RMount/LConn1
  Rigid Transform/LConn1 -- Y-Axis Unit/LConn2
  X-Axis Unit1/LConn2 -- YMount1/RConn1
  Rigid Transform2/LConn1 -- Z-Axis Unit/LConn2
  YMount2/RConn1 -- X-Axis Unit2/LConn2
  YMount2/LConn1 -- Y-Axis Unit/RConn2
  Structure2/RConn1 -- B/RConn1 -- Structure1/RConn1
  Structure1/LConn1 -- X-Axis Unit1/RConn1
  Structure2/LConn1 -- X-Axis Unit2/RConn1
  Z-Axis Unit/RConn1 -- Rigid Transform1/RConn1
  ZMount/RConn1 -- Rigid Transform/RConn1
  Y-Axis Unit/RConn1 -- YMount1/LConn1
  Rigid Transform1/LConn1 -- ZMount/LConn1
  RA/RConn1 -- R-Axis Unit/LConn2
  R-Axis Unit/LConn1 -- Rigid Transform4/RConn1
  F/RConn1 -- R-Axis Unit/RConn1

== system GantryRobotSubsystem/GantryRobotVariant/XY Gantry/Structure1 ==
  Column1 : CartesianLib/Column  lengthColumn=heightColumn  widthColumn=widthColumn  typeInertiaColumn=Calculate from Geometry  densityColumn=7780  massColumn=1  CMColumn=[0 0 0]  MOIColumn=[1 1 1]  POIColumn=[0 0 0]  colorColumn=[0.8 0.2 0.2]
  Column2 : CartesianLib/Column  lengthColumn=heightColumn  widthColumn=widthColumn  typeInertiaColumn=Calculate from Geometry  densityColumn=7780  massColumn=1  CMColumn=[0 0 0]  MOIColumn=[1 1 1]  POIColumn=[0 0 0]  colorColumn=[0.8 0.2 0.2]
  Rigid Transform1 : sm_lib/Frames and Transforms/Rigid Transform  RotationMethod=None  FollAlignAxisA=+X  BaseAlignAxisA=+Y  FollAlignAxisB=+Y  BaseAlignAxisB=+Z  RotationStandardAxis=+Z  RotationAngle=0  RotationAngleUnits=deg  RotationArbitraryAxis=[0 0 1]  RotationSequenceAxes=FollowerAxes  RotationSequence=XYX  RotationSequenceAngles=[0 0 0]  RotationSequenceAnglesUnits=deg  RotationMatrix=[1 0 0;0 1 0;0 0 1]  Quaternion=[1 0 0 0]  TranslationMethod=Cartesian  TranslationCartesianOffset=positionColumn1  TranslationCartesianOffsetUnits=m  TranslationStandardAxis=+Z  TranslationStandardOffset=0  TranslationStandardOffsetUnits=m  TranslationROffset=0  TranslationROffsetUnits=m  TranslationThetaOffset=0  TranslationThetaOffsetUnits=deg  TranslationZOffset=0  TranslationZOffsetUnits=m
  Rigid Transform2 : sm_lib/Frames and Transforms/Rigid Transform  RotationMethod=None  FollAlignAxisA=+X  BaseAlignAxisA=+Y  FollAlignAxisB=+Y  BaseAlignAxisB=+Z  RotationStandardAxis=+Z  RotationAngle=0  RotationAngleUnits=deg  RotationArbitraryAxis=[0 0 1]  RotationSequenceAxes=FollowerAxes  RotationSequence=XYX  RotationSequenceAngles=[0 0 0]  RotationSequenceAnglesUnits=deg  RotationMatrix=[1 0 0;0 1 0;0 0 1]  Quaternion=[1 0 0 0]  TranslationMethod=Cartesian  TranslationCartesianOffset=positionColumn2  TranslationCartesianOffsetUnits=m  TranslationStandardAxis=+Z  TranslationStandardOffset=0  TranslationStandardOffsetUnits=m  TranslationROffset=0  TranslationROffsetUnits=m  TranslationThetaOffset=0  TranslationThetaOffsetUnits=deg  TranslationZOffset=0  TranslationZOffsetUnits=m
  Weld Joint : sm_lib/Joints/Weld Joint  JointMode=Normal  CompositeWrenchDir=FollowerOnBase  CompositeWrenchFrame=BaseFrame  SenseConstraintForce=off  SenseConstraintTorque=off  SenseTotalForce=off  SenseTotalTorque=off
  Weld Joint1 : sm_lib/Joints/Weld Joint  JointMode=Normal  CompositeWrenchDir=FollowerOnBase  CompositeWrenchFrame=BaseFrame  SenseConstraintForce=off  SenseConstraintTorque=off  SenseTotalForce=off  SenseTotalTorque=off
  XMount1 : CartesianLib/Mount  typeMount=Plate mount  widthMount=widthXMount  angleMount=45  angleRotate=0  typeInertiaMount=Calculate from Geometry  densityMount=7780  massMount=0.1  CMMount=[0 0 0]  MOIMount=[1 1 1]  POIMount=[0 0 0]  colorMount=[0.35 0.25 0.25]
  XMount2 : CartesianLib/Mount  typeMount=Plate mount  widthMount=widthXMount  angleMount=45  angleRotate=0  typeInertiaMount=Calculate from Geometry  densityMount=7780  massMount=0.1  CMMount=[0 0 0]  MOIMount=[1 1 1]  POIMount=[0 0 0]  colorMount=[0.35 0.25 0.25]
  F1 : PMIOPort  Side=Left
  B : PMIOPort  Port=2  Side=Right
  F2 : PMIOPort  Port=3  Side=Left
  connections:
  Weld Joint1/RConn1 -- Column2/RConn1
  Rigid Transform2/RConn1 -- Weld Joint1/LConn1
  Rigid Transform1/RConn1 -- Weld Joint/LConn1
  B/RConn1 -- Rigid Transform2/LConn1 -- Rigid Transform1/LConn1
  F2/RConn1 -- XMount2/LConn1
  XMount2/RConn1 -- Column2/LConn1
  Column1/LConn1 -- XMount1/RConn1
  XMount1/LConn1 -- F1/RConn1
  Weld Joint/RConn1 -- Column1/RConn1

== system GantryRobotSubsystem/GantryRobotVariant/XY Gantry/Structure2 ==
  Column3 : CartesianLib/Column  lengthColumn=heightColumn  widthColumn=widthColumn  typeInertiaColumn=Calculate from Geometry  densityColumn=7780  massColumn=1  CMColumn=[0 0 0]  MOIColumn=[1 1 1]  POIColumn=[0 0 0]  colorColumn=[0.8 0.2 0.2]
  Column4 : CartesianLib/Column  lengthColumn=heightColumn  widthColumn=widthColumn  typeInertiaColumn=Calculate from Geometry  densityColumn=7780  massColumn=1  CMColumn=[0 0 0]  MOIColumn=[1 1 1]  POIColumn=[0 0 0]  colorColumn=[0.8 0.2 0.2]
  Rigid Transform1 : sm_lib/Frames and Transforms/Rigid Transform  RotationMethod=None  FollAlignAxisA=+X  BaseAlignAxisA=+Y  FollAlignAxisB=+Y  BaseAlignAxisB=+Z  RotationStandardAxis=+Z  RotationAngle=0  RotationAngleUnits=deg  RotationArbitraryAxis=[0 0 1]  RotationSequenceAxes=FollowerAxes  RotationSequence=XYX  RotationSequenceAngles=[0 0 0]  RotationSequenceAnglesUnits=deg  RotationMatrix=[1 0 0;0 1 0;0 0 1]  Quaternion=[1 0 0 0]  TranslationMethod=Cartesian  TranslationCartesianOffset=positionColumn3  TranslationCartesianOffsetUnits=m  TranslationStandardAxis=+Z  TranslationStandardOffset=0  TranslationStandardOffsetUnits=m  TranslationROffset=0  TranslationROffsetUnits=m  TranslationThetaOffset=0  TranslationThetaOffsetUnits=deg  TranslationZOffset=0  TranslationZOffsetUnits=m
  Rigid Transform2 : sm_lib/Frames and Transforms/Rigid Transform  RotationMethod=None  FollAlignAxisA=+X  BaseAlignAxisA=+Y  FollAlignAxisB=+Y  BaseAlignAxisB=+Z  RotationStandardAxis=+Z  RotationAngle=0  RotationAngleUnits=deg  RotationArbitraryAxis=[0 0 1]  RotationSequenceAxes=FollowerAxes  RotationSequence=XYX  RotationSequenceAngles=[0 0 0]  RotationSequenceAnglesUnits=deg  RotationMatrix=[1 0 0;0 1 0;0 0 1]  Quaternion=[1 0 0 0]  TranslationMethod=Cartesian  TranslationCartesianOffset=positionColumn4  TranslationCartesianOffsetUnits=m  TranslationStandardAxis=+Z  TranslationStandardOffset=0  TranslationStandardOffsetUnits=m  TranslationROffset=0  TranslationROffsetUnits=m  TranslationThetaOffset=0  TranslationThetaOffsetUnits=deg  TranslationZOffset=0  TranslationZOffsetUnits=m
  Weld Joint : sm_lib/Joints/Weld Joint  JointMode=Normal  CompositeWrenchDir=FollowerOnBase  CompositeWrenchFrame=BaseFrame  SenseConstraintForce=off  SenseConstraintTorque=off  SenseTotalForce=off  SenseTotalTorque=off
  Weld Joint1 : sm_lib/Joints/Weld Joint  JointMode=Normal  CompositeWrenchDir=FollowerOnBase  CompositeWrenchFrame=BaseFrame  SenseConstraintForce=off  SenseConstraintTorque=off  SenseTotalForce=off  SenseTotalTorque=off
  XMount3 : CartesianLib/Mount  typeMount=Plate mount  widthMount=widthXMount  angleMount=45  angleRotate=0  typeInertiaMount=Calculate from Geometry  densityMount=7780  massMount=0.1  CMMount=[0 0 0]  MOIMount=[1 1 1]  POIMount=[0 0 0]  colorMount=[0.35 0.25 0.25]
  XMount4 : CartesianLib/Mount  typeMount=Plate mount  widthMount=widthXMount  angleMount=45  angleRotate=0  typeInertiaMount=Calculate from Geometry  densityMount=7780  massMount=0.1  CMMount=[0 0 0]  MOIMount=[1 1 1]  POIMount=[0 0 0]  colorMount=[0.35 0.25 0.25]
  F1 : PMIOPort  Side=Left
  B : PMIOPort  Port=2  Side=Right
  F2 : PMIOPort  Port=3  Side=Left
  connections:
  Weld Joint1/RConn1 -- Column4/RConn1
  Weld Joint/RConn1 -- Column3/RConn1
  Rigid Transform2/RConn1 -- Weld Joint1/LConn1
  Rigid Transform1/RConn1 -- Weld Joint/LConn1
  B/RConn1 -- Rigid Transform2/LConn1 -- Rigid Transform1/LConn1
  F2/RConn1 -- XMount4/LConn1
  Column3/LConn1 -- XMount3/RConn1
  XMount3/LConn1 -- F1/RConn1
  XMount4/RConn1 -- Column4/LConn1

== system GantryRobotSubsystem/GantryRobotVariant/XY Gantry/Subsystem ==
  note: Dummy ZS signals
  Constant : Constant  Value=0
  Constant1 : Constant  Value=0
  Constant2 : Constant  Value=0
  Bus Element Out : Outport  PortName=ZS  Element=Zp (m)
  BusElementOut : Outport  PortName=ZS  Element=Zv (m/s)
  BusElementOut1 : Outport  PortName=ZS  Element=Za (m^2/s)
  wires:
  Constant/1 -> Bus Element Out/1
  Constant1/1 -> BusElementOut/1
  Constant2/1 -> BusElementOut1/1

== system GantryRobotSubsystem/GantryRobotVariant/XY Gantry/Subsystem1 ==
  note: Dummy RS signals
  Constant : Constant  Value=0
  Constant1 : Constant  Value=0
  Bus Element Out : Outport  PortName=RS  Element=q (rad)
  BusElementOut : Outport  PortName=RS  Element=w (rad/s)
  wires:
  Constant/1 -> Bus Element Out/1
  Constant1/1 -> BusElementOut/1
